simulink model "iot_casestudy_1_32"  (R2023a)
settings: Solver=VariableStepAuto  StartTime=0.0  StopTime=3.0  RelTol=1e-3
undefined symbols (not defined in the file or in its folder): m, n
(part 3 of 3)

== stateflow chart iot_casestudy_1_32/CameraScheduler29 ==
  settings: updateMethod=CONTINUOUS  executeAtInitialization=1
  state Main
    entry:
    dt=timer_array[i];
  (default) -> Main : {i=0;dt=0;}
  Main -> Main : after(dt,msec){i=i+1;send(schedule_driver);send(schedule_control);}
  data: timer_array input; i local double; schedule_driver output double; schedule_control output double; dt local double

== stateflow chart iot_casestudy_1_32/CameraScheduler30 ==
  settings: updateMethod=CONTINUOUS  executeAtInitialization=1
  state Main
    entry:
    dt=timer_array[i];
  (default) -> Main : {i=1;dt=0;}
  Main -> Main : after(dt,msec){i=i+1;send(schedule_driver);send(schedule_control);}
  data: timer_array input; schedule_driver output double; schedule_control output double; dt local double; dt2 local double; i local double =0.0

== stateflow chart iot_casestudy_1_32/CameraScheduler31 ==
  settings: updateMethod=CONTINUOUS  executeAtInitialization=1
  state Main
    entry:
    dt=timer_array[i];
  (default) -> Main : {i=0;dt=0;}
  Main -> Main : after(dt,msec){i=i+1;send(schedule_driver);send(schedule_control);}
  data: timer_array input; i local double; schedule_driver output double; schedule_control output double; dt local double

== stateflow chart iot_casestudy_1_32/CameraDriver ==
  settings: updateMethod=CONTINUOUS
  state Operation
    state CarVisibility [parallel]
      settings: executionOrder=1
      state NoCar
        entry: car=0;
      state Car
        entry: car=1;
      (default) -> NoCar
      NoCar -> Car : [traffic_state==1]
      Car -> NoCar : [traffic_state==0]
    state DriverOperation [parallel]
      settings: executionOrder=2
      state Main
      (default) -> Main : {i=1;}
      Main -> (junction 22) : schedule[image_request]
      (junction 22) -> Main [order 2] : {image.data=0;
          | send(image);i = i + 1;}
      (junction 22) -> Main [order 1] : [(car==1)&&(blurryness(i)==1)]
          | {image.data=1;i = i + 1;send(image);}
  data: image_request input; traffic_state input; blurryness input; image output; car local; i local; schedule input

== stateflow chart iot_casestudy_1_32/CameraControl ==
  settings: updateMethod=CONTINUOUS
  state Operation
    state RequestHangling [parallel]
      settings: executionOrder=1
      state Operation1
      (default) -> Operation1 : {image_request=1;}
      Operation1 -> Operation1 : schedule{image_request=1;}
    state ImageMessaging [parallel]
      settings: executionOrder=2
      state Operation2
        entry:
        validity=isvalid(imageIn);
      (default) -> Operation2 : {i=1;}
      (junction 28) -> Operation2 [order 1] : [validity==1]
          | {receive(imageIn);i = i + 1;
          | imageOut.data=imageIn.data
          | send(imageOut);}
      (junction 28) -> Operation2 [order 2] : {i = i + 1;receive(imageIn);}
      (junction 19) -> (junction 28) [order 1] : [network_faults(i)==0]
      (junction 19) -> Operation2 [order 2] : {receive(imageIn);i = i + 1;}
      Operation2 -> (junction 19) : schedule
  (default) -> Operation
  data: image_request output; imageIn input; i local; network_faults input; imageOut output; schedule input; validity local

== stateflow chart iot_casestudy_1_32/Traffic ==
  settings: updateMethod=CONTINUOUS
  state Nocar
    entry:
    traffic_state=0;
  state Car
    entry:
    traffic_state=1;
  state Nocar1
    entry:
    traffic_state=0;
  (default) -> Nocar
  Nocar -> Car : after(arrive_time,msec)
  Car -> Nocar1 : after(visibility_time,msec)
  data: arrive_time input; visibility_time input; traffic_state output

== stateflow chart iot_casestudy_1_32/Edge ==
  state Waiting
  state NotRecognized
    wait_time=elapsed(msec);
  state Recognized
  (default) -> Waiting : {faults=0;}
  Waiting -> Waiting [order 5] : image3{receive(image3);}
  Waiting -> Waiting [order 3] : image1{receive(image1);}
  Waiting -> Waiting [order 6] : image4{receive(image4);}
  Waiting -> Waiting [order 18] : image17{receive(image17);}
  Waiting -> Waiting [order 19] : image18{receive(image18);}
  Waiting -> Waiting [order 26] : image25{receive(image25);}
  Waiting -> Waiting [order 7] : image5{receive(image5);}
  Waiting -> Waiting [order 9] : image8{receive(image8);}
  Waiting -> Waiting [order 21] : image20{receive(image20);}
  Waiting -> Waiting [order 29] : image28{receive(image28);}
  Waiting -> Waiting [order 20] : image19{receive(image19);}
  Waiting -> Waiting [order 23] : image22{receive(image22);}
  Waiting -> Waiting [order 25] : image24{receive(image24);}
  Waiting -> Waiting [order 2] : image2{receive(image2);}
  Waiting -> Waiting [order 22] : image21{receive(image21);}
  Waiting -> Waiting [order 24] : image23{receive(image23);}
  Waiting -> Waiting [order 32] : image31{receive(image31);}
  Waiting -> Waiting [order 1] : image6{receive(image6);}
  Waiting -> Waiting [order 27] : image26{receive(image26);}
  Waiting -> Waiting [order 33] : image32{receive(image32);}
  Waiting -> Waiting [order 31] : image30{receive(image30);}
  Waiting -> Waiting [order 8] : image7{receive(image7);}
  Waiting -> Waiting [order 28] : image27{receive(image27);}
  Waiting -> Waiting [order 30] : image29{receive(image29);}
  Recognized -> Waiting [order 1] : [traffic_state==0]
  Waiting -> NotRecognized [order 4] : [traffic_state==1]
  NotRecognized -> Waiting [order 1] : [traffic_state==0]
      | {faults=1;}
  Waiting -> Waiting [order 10] : image9{receive(image9);}
  Waiting -> Waiting [order 11] : image10{receive(image10);}
  Waiting -> Waiting [order 12] : image11{receive(image11);}
  Waiting -> Waiting [order 13] : image12{receive(image12);}
  Waiting -> Waiting [order 14] : image13{receive(image13);}
  Waiting -> Waiting [order 15] : image14{receive(image14);}
  Waiting -> Waiting [order 16] : image15{receive(image15);}
  Waiting -> Waiting [order 17] : image16{receive(image16);}
  (junction 279) -> NotRecognized [order 2]
  NotRecognized -> (junction 279) [order 19] : image32
      | {receive(image32);}
  (junction 284) -> NotRecognized [order 2]
  NotRecognized -> (junction 284) [order 18] : image31
      | {receive(image31);}
  (junction 277) -> NotRecognized [order 2]
  NotRecognized -> (junction 277) [order 17] : image30
      | {receive(image30);}
  (junction 276) -> NotRecognized [order 2]
  NotRecognized -> (junction 276) [order 15] : image29
      | {receive(image29);}
  (junction 305) -> NotRecognized [order 2]
  NotRecognized -> (junction 305) [order 13] : image28
      | {receive(image28);}
  (junction 263) -> NotRecognized [order 2]
  NotRecognized -> (junction 263) [order 11] : image27
      | {receive(image27);}
  (junction 303) -> NotRecognized [order 2]
  NotRecognized -> (junction 303) [order 9] : image26
      | {receive(image26);}
  (junction 285) -> NotRecognized [order 2]
  NotRecognized -> (junction 285) [order 7] : image25
      | {receive(image25);}
  (junction 302) -> NotRecognized [order 2]
  NotRecognized -> (junction 302) [order 16] : image24
      | {receive(image24);}
  (junction 297) -> NotRecognized [order 2]
  NotRecognized -> (junction 297) [order 14] : image23
      | {receive(image23);}
  (junction 287) -> NotRecognized [order 2]
  NotRecognized -> (junction 287) [order 12] : image22
      | {receive(image22);}
  (junction 318) -> NotRecognized [order 2]
  NotRecognized -> (junction 318) [order 10] : image21
      | {receive(image21);}
  (junction 264) -> NotRecognized [order 2]
  NotRecognized -> (junction 264) [order 8] : image20
      | {receive(image20);}
  (junction 269) -> NotRecognized [order 2]
  NotRecognized -> (junction 269) [order 6] : image19
      | {receive(image19);}
  (junction 261) -> NotRecognized [order 2]
  NotRecognized -> (junction 261) [order 4] : image18
      | {receive(image18);}
  (junction 272) -> NotRecognized [order 2]
  NotRecognized -> (junction 272) [order 3] : image17
      | {receive(image17);}
  (junction 119) -> NotRecognized [order 2]
  NotRecognized -> (junction 119) [order 5] : image16
      | {receive(image16);}
  (junction 117) -> NotRecognized [order 2]
  NotRecognized -> (junction 117) [order 20] : image15
      | {receive(image15);}
  (junction 106) -> NotRecognized [order 2]
  NotRecognized -> (junction 106) [order 21] : image14
      | {receive(image14);}
  (junction 132) -> NotRecognized [order 2]
  NotRecognized -> (junction 132) [order 22] : image13
      | {receive(image13);}
  (junction 108) -> NotRecognized [order 2]
  NotRecognized -> (junction 108) [order 23] : image12
      | {receive(image12);}
  (junction 113) -> NotRecognized [order 2]
  NotRecognized -> (junction 113) [order 24] : image11
      | {receive(image11);}
  (junction 105) -> NotRecognized [order 2]
  NotRecognized -> (junction 105) [order 25] : image10
      | {receive(image10);}
  (junction 120) -> NotRecognized [order 2]
  NotRecognized -> (junction 120) [order 27] : image9
      | {receive(image9);}
  (junction 64) -> NotRecognized [order 2]
  NotRecognized -> (junction 64) [order 33] : image8
      | {receive(image8);}
  (junction 63) -> NotRecognized [order 2]
  NotRecognized -> (junction 63) [order 32] : image7
      | {receive(image7);}
  (junction 62) -> NotRecognized [order 2]
  NotRecognized -> (junction 62) [order 31] : image6
      | {receive(image6);}
  (junction 61) -> NotRecognized [order 2]
  NotRecognized -> (junction 61) [order 30] : image5
      | {receive(image5);}
  (junction 49) -> NotRecognized [order 2]
  NotRecognized -> (junction 49) [order 29] : image4
      | {receive(image4);}
  (junction 45) -> NotRecognized [order 2]
  NotRecognized -> (junction 45) [order 28] : image3
      | {receive(image3);}
  (junction 22) -> NotRecognized [order 2]
  NotRecognized -> (junction 22) [order 2] : image2
      | {receive(image2);}
  (junction 10) -> NotRecognized [order 2]
  NotRecognized -> (junction 10) [order 26] : image1{receive(image1);}
  (junction 264) -> Recognized [order 1] : [image20.data==1]
  (junction 261) -> Recognized [order 1] : [image18.data==1]
  (junction 49) -> Recognized [order 1] : [image4.data==1]
  (junction 22) -> Recognized [order 1] : [image2.data==1]
  (junction 302) -> Recognized [order 1] : [image24.data==1]
  (junction 287) -> Recognized [order 1] : [image22.data==1]
  (junction 64) -> Recognized [order 1] : [image8.data==1]
  (junction 62) -> Recognized [order 1] : [image6.data==1]
  (junction 279) -> Recognized [order 1] : [image32.data==1]
  (junction 305) -> Recognized [order 1] : [image28.data==1]
  (junction 303) -> Recognized [order 1] : [image26.data==1]
  (junction 119) -> Recognized [order 1] : [image16.data==1]
  (junction 108) -> Recognized [order 1] : [image12.data==1]
  (junction 105) -> Recognized [order 1] : [image10.data==1]
  (junction 277) -> Recognized [order 1] : [image30.data==1]
  (junction 106) -> Recognized [order 1] : [image14.data==1]
  Recognized -> Recognized [order 2] : image17{receive(image17);}
  Recognized -> Recognized [order 29] : image18{receive(image18);}
  Recognized -> Recognized [order 31] : image20{receive(image20);}
  Recognized -> Recognized [order 10] : image25{receive(image25);}
  Recognized -> Recognized [order 30] : image19{receive(image19);}
  Recognized -> Recognized [order 32] : image21{receive(image21);}
  Recognized -> Recognized [order 11] : image24{receive(image24);}
  Recognized -> Recognized [order 3] : image32{receive(image32);}
  Recognized -> Recognized [order 33] : image22{receive(image22);}
  Recognized -> Recognized [order 7] : image28{receive(image28);}
  Recognized -> Recognized [order 4] : image31{receive(image31);}
  Recognized -> Recognized [order 5] : image30{receive(image30);}
  Recognized -> Recognized [order 12] : image23{receive(image23);}
  Recognized -> Recognized [order 9] : image26{receive(image26);}
  Recognized -> Recognized [order 8] : image27{receive(image27);}
  Recognized -> Recognized [order 6] : image29{receive(image29);}
  (junction 10) -> Recognized [order 1] : [image1.data==1]
  (junction 263) -> Recognized [order 1] : [image27.data==1]
  (junction 285) -> Recognized [order 1] : [image25.data==1]
  (junction 297) -> Recognized [order 1] : [image23.data==1]
  (junction 318) -> Recognized [order 1] : [image21.data==1]
  (junction 269) -> Recognized [order 1] : [image19.data==1]
  (junction 272) -> Recognized [order 1] : [image17.data==1]
  (junction 113) -> Recognized [order 1] : [image11.data==1]
  (junction 120) -> Recognized [order 1] : [image9.data==1]
  (junction 63) -> Recognized [order 1] : [image7.data==1]
  (junction 61) -> Recognized [order 1] : [image5.data==1]
  (junction 45) -> Recognized [order 1] : [image3.data==1]
  (junction 284) -> Recognized [order 1] : [image31.data==1]
  (junction 276) -> Recognized [order 1] : [image29.data==1]
  (junction 117) -> Recognized [order 1] : [image15.data==1]
  (junction 132) -> Recognized [order 1] : [image13.data==1]
  Recognized -> Recognized [order 21] : image9{receive(image9);}
  Recognized -> Recognized [order 22] : image10{receive(image10);}
  Recognized -> Recognized [order 23] : image11{receive(image11);}
  Recognized -> Recognized [order 24] : image12{receive(image12);}
  Recognized -> Recognized [order 25] : image13{receive(image13);}
  Recognized -> Recognized [order 26] : image14{receive(image14);}
  Recognized -> Recognized [order 27] : image15{receive(image15);}
  Recognized -> Recognized [order 28] : image16{receive(image16);}
  Recognized -> Recognized [order 17] : image8{receive(image8);}
  Recognized -> Recognized [order 18] : image7{receive(image7);}
  Recognized -> Recognized [order 19] : image6{receive(image6);}
  Recognized -> Recognized [order 20] : image5{receive(image5);}
  Recognized -> Recognized [order 13] : image3{receive(image3);}
  Recognized -> Recognized [order 16] : image4{receive(image4);}
  Recognized -> Recognized [order 14] : image2{receive(image2);}
  Recognized -> Recognized [order 15] : image1{receive(image1);}
  data: traffic_state input; image1 input; faults output; image2 input; wait_time output; image3 input; image4 input; image5 input; image6 input; image7 input; image8 input; image9 input; image10 input; image11 input; image12 input; image13 input; image14 input; image15 input; image16 input; image17 input; image18 input; image19 input; image20 input; image21 input; image22 input; image23 input; image24 input; image25 input; image26 input; image27 input; image28 input; image29 input; image30 input; image31 input; image32 input

== stateflow chart iot_casestudy_1_32/CameraScheduler ==
  settings: updateMethod=CONTINUOUS  executeAtInitialization=1
  state Main
    entry:
    dt=timer_array[i];
  (default) -> Main : {i=1;dt=0;}
  Main -> Main : after(dt,msec){i=i+1;send(schedule_driver);send(schedule_control);}
  data: timer_array input; schedule_driver output double; schedule_control output double; dt local double; dt2 local double; i output double =0.0

== stateflow chart iot_casestudy_1_32/CameraControl1 ==
  settings: updateMethod=CONTINUOUS
  state Operation
    state RequestHangling [parallel]
      settings: executionOrder=1
      note: {image_request=1;}
      state Operation1
      (default) -> Operation1
      Operation1 -> Operation1 : schedule{image_request=1;}
    state ImageMessaging [parallel]
      settings: executionOrder=2
      state Operation2
        entry:
        validity=isvalid(imageIn);
      (default) -> Operation2 : {i=1;}
      (junction 29) -> Operation2 [order 1] : [isvalid(imageIn)==1]
          | {receive(imageIn);i = i + 1;
          | imageOut.data=imageIn.data;
          | send(imageOut);}
      (junction 19) -> Operation2 [order 2] : {receive(imageIn);i = i + 1;}
      Operation2 -> (junction 19) : schedule
      (junction 29) -> Operation2 [order 2] : {i = i + 1;receive(imageIn);}
      (junction 19) -> (junction 29) [order 1] : [network_faults(i)==0]
  (default) -> Operation
  data: image_request output; imageIn input; i local; network_faults input; imageOut output; schedule input; validity local

== stateflow chart iot_casestudy_1_32/CameraDriver1 ==
  settings: updateMethod=CONTINUOUS
  state Operation
    state CarVisibility [parallel]
      settings: executionOrder=1
      state NoCar
        entry: car=0;
      state Car
        entry: car=1;
      (default) -> NoCar
      NoCar -> Car : [traffic_state==1]
      Car -> NoCar : [traffic_state==0]
    state DriverOperation [parallel]
      settings: executionOrder=2
      state Main
      (default) -> Main : {i=1;}
      Main -> (junction 22) : schedule
          | [image_request]
      (junction 22) -> Main [order 1] : [(car==1)&&(blurryness(i)==1)]
          | {image.data=1;send(image);i = i + 1;}
      (junction 22) -> Main [order 2] : {image.data=0;
          | send(image);i = i + 1;}
  data: image_request input; traffic_state input; blurryness input; image output; car local; i local; schedule input

== stateflow chart iot_casestudy_1_32/CameraScheduler1 ==
  settings: updateMethod=CONTINUOUS  executeAtInitialization=1
  state Main
    entry:
    dt=timer_array[i];
  (default) -> Main : {i=0;dt=0;}
  Main -> Main : after(dt,msec){i=i+1;send(schedule_driver);send(schedule_control);}
  data: timer_array input; i local double; schedule_driver output double; schedule_control output double; dt local double

== stateflow chart iot_casestudy_1_32/CameraControl2 ==
  settings: updateMethod=CONTINUOUS
  state Operation
    state RequestHangling [parallel]
      settings: executionOrder=1
      state Operation1
      (default) -> Operation1 : {image_request=1;}
      Operation1 -> Operation1 : schedule{image_request=1;}
    state ImageMessaging [parallel]
      settings: executionOrder=2
      state Operation2
        entry:
        validity=isvalid(imageIn);
      (default) -> Operation2 : {i=1;}
      (junction 28) -> Operation2 [order 1] : [validity==1]
          | {receive(imageIn);i = i + 1;
          | imageOut.data=imageIn.data
          | send(imageOut);}
      (junction 28) -> Operation2 [order 2] : {i = i + 1;receive(imageIn);}
      (junction 19) -> (junction 28) [order 1] : [network_faults(i)==0]
      (junction 19) -> Operation2 [order 2] : {receive(imageIn);i = i + 1;}
      Operation2 -> (junction 19) : schedule
  (default) -> Operation
  data: image_request output; imageIn input; i local; network_faults input; imageOut output; schedule input; validity local

== stateflow chart iot_casestudy_1_32/CameraControl3 ==
  settings: updateMethod=CONTINUOUS
  state Operation
    state RequestHangling [parallel]
      settings: executionOrder=1
      note: {image_request=1;}
      state Operation1
      (default) -> Operation1
      Operation1 -> Operation1 : schedule{image_request=1;}
    state ImageMessaging [parallel]
      settings: executionOrder=2
      state Operation2
        entry:
        validity=isvalid(imageIn);
      (default) -> Operation2 : {i=1;}
      (junction 29) -> Operation2 [order 1] : [isvalid(imageIn)==1]
          | {receive(imageIn);i = i + 1;
          | imageOut.data=imageIn.data;
          | send(imageOut);}
      (junction 19) -> Operation2 [order 2] : {receive(imageIn);i = i + 1;}
      Operation2 -> (junction 19) : schedule
      (junction 29) -> Operation2 [order 2] : {i = i + 1;receive(imageIn);}
      (junction 19) -> (junction 29) [order 1] : [network_faults(i)==0]
  (default) -> Operation
  data: image_request output; imageIn input; i local; network_faults input; imageOut output; schedule input; validity local

== stateflow chart iot_casestudy_1_32/CameraDriver2 ==
  settings: updateMethod=CONTINUOUS
  state Operation
    state CarVisibility [parallel]
      settings: executionOrder=1
      state NoCar
        entry: car=0;
      state Car
        entry: car=1;
      (default) -> NoCar
      NoCar -> Car : [traffic_state==1]
      Car -> NoCar : [traffic_state==0]
    state DriverOperation [parallel]
      settings: executionOrder=2
      state Main
      (default) -> Main : {i=1;}
      Main -> (junction 22) : schedule[image_request]
      (junction 22) -> Main [order 2] : {image.data=0;
          | send(image);i = i + 1;}
      (junction 22) -> Main [order 1] : [(car==1)&&(blurryness(i)==1)]
          | {image.data=1;i = i + 1;send(image);}
  data: image_request input; traffic_state input; blurryness input; image output; car local; i local; schedule input

== stateflow chart iot_casestudy_1_32/CameraDriver3 ==
  settings: updateMethod=CONTINUOUS
  state Operation
    state CarVisibility [parallel]
      settings: executionOrder=1
      state NoCar
        entry: car=0;
      state Car
        entry: car=1;
      (default) -> NoCar
      NoCar -> Car : [traffic_state==1]
      Car -> NoCar : [traffic_state==0]
    state DriverOperation [parallel]
      settings: executionOrder=2
      state Main
      (default) -> Main : {i=1;}
      Main -> (junction 22) : schedule
          | [image_request]
      (junction 22) -> Main [order 1] : [(car==1)&&(blurryness(i)==1)]
          | {image.data=1;send(image);i = i + 1;}
      (junction 22) -> Main [order 2] : {image.data=0;
          | send(image);i = i + 1;}
  data: image_request input; traffic_state input; blurryness input; image output; car local; i local; schedule input

== stateflow chart iot_casestudy_1_32/CameraScheduler2 ==
  settings: updateMethod=CONTINUOUS  executeAtInitialization=1
  state Main
    entry:
    dt=timer_array[i];
  (default) -> Main : {i=1;dt=0;}
  Main -> Main : after(dt,msec){i=i+1;send(schedule_driver);send(schedule_control);}
  data: timer_array input; schedule_driver output double; schedule_control output double; dt local double; dt2 local double; i output double =0.0

== stateflow chart iot_casestudy_1_32/CameraScheduler3 ==
  settings: updateMethod=CONTINUOUS  executeAtInitialization=1
  state Main
    entry:
    dt=timer_array[i];
  (default) -> Main : {i=0;dt=0;}
  Main -> Main : after(dt,msec){i=i+1;send(schedule_driver);send(schedule_control);}
  data: timer_array input; i local double; schedule_driver output double; schedule_control output double; dt local double

== stateflow chart iot_casestudy_1_32/CameraControl4 ==
  settings: updateMethod=CONTINUOUS
  state Operation
    state RequestHangling [parallel]
      settings: executionOrder=1
      state Operation1
      (default) -> Operation1 : {image_request=1;}
      Operation1 -> Operation1 : schedule{image_request=1;}
    state ImageMessaging [parallel]
      settings: executionOrder=2
      state Operation2
        entry:
        validity=isvalid(imageIn);
      (default) -> Operation2 : {i=1;}
      (junction 28) -> Operation2 [order 1] : [validity==1]
          | {receive(imageIn);i = i + 1;
          | imageOut.data=imageIn.data
          | send(imageOut);}
      (junction 28) -> Operation2 [order 2] : {i = i + 1;receive(imageIn);}
      (junction 19) -> (junction 28) [order 1] : [network_faults(i)==0]
      (junction 19) -> Operation2 [order 2] : {receive(imageIn);i = i + 1;}
      Operation2 -> (junction 19) : schedule
  (default) -> Operation
  data: image_request output; imageIn input; i local; network_faults input; imageOut output; schedule input; validity local

== stateflow chart iot_casestudy_1_32/CameraControl5 ==
  settings: updateMethod=CONTINUOUS
  state Operation
    state RequestHangling [parallel]
      settings: executionOrder=1
      note: {image_request=1;}
      state Operation1
      (default) -> Operation1
      Operation1 -> Operation1 : schedule{image_request=1;}
    state ImageMessaging [parallel]
      settings: executionOrder=2
      state Operation2
        entry:
        validity=isvalid(imageIn);
      (default) -> Operation2 : {i=1;}
      (junction 29) -> Operation2 [order 1] : [isvalid(imageIn)==1]
          | {receive(imageIn);i = i + 1;
          | imageOut.data=imageIn.data;
          | send(imageOut);}
      (junction 19) -> Operation2 [order 2] : {receive(imageIn);i = i + 1;}
      Operation2 -> (junction 19) : schedule
      (junction 29) -> Operation2 [order 2] : {i = i + 1;receive(imageIn);}
      (junction 19) -> (junction 29) [order 1] : [network_faults(i)==0]
  (default) -> Operation
  data: image_request output; imageIn input; i local; network_faults input; imageOut output; schedule input; validity local

== stateflow chart iot_casestudy_1_32/CameraControl6 ==
  settings: updateMethod=CONTINUOUS
  state Operation
    state RequestHangling [parallel]
      settings: executionOrder=1
      state Operation1
      (default) -> Operation1 : {image_request=1;}
      Operation1 -> Operation1 : schedule{image_request=1;}
    state ImageMessaging [parallel]
      settings: executionOrder=2
      state Operation2
        entry:
        validity=isvalid(imageIn);
      (default) -> Operation2 : {i=1;}
      (junction 28) -> Operation2 [order 1] : [validity==1]
          | {receive(imageIn);i = i + 1;
          | imageOut.data=imageIn.data
          | send(imageOut);}
      (junction 28) -> Operation2 [order 2] : {i = i + 1;receive(imageIn);}
      (junction 19) -> (junction 28) [order 1] : [network_faults(i)==0]
      (junction 19) -> Operation2 [order 2] : {receive(imageIn);i = i + 1;}
      Operation2 -> (junction 19) : schedule
  (default) -> Operation
  data: image_request output; imageIn input; i local; network_faults input; imageOut output; schedule input; validity local

== stateflow chart iot_casestudy_1_32/CameraControl7 ==
  settings: updateMethod=CONTINUOUS
  state Operation
    state RequestHangling [parallel]
      settings: executionOrder=1
      note: {image_request=1;}
      state Operation1
      (default) -> Operation1
      Operation1 -> Operation1 : schedule{image_request=1;}
    state ImageMessaging [parallel]
      settings: executionOrder=2
      state Operation2
        entry:
        validity=isvalid(imageIn);
      (default) -> Operation2 : {i=1;}
      (junction 29) -> Operation2 [order 1] : [isvalid(imageIn)==1]
          | {receive(imageIn);i = i + 1;
          | imageOut.data=imageIn.data;
          | send(imageOut);}
      (junction 19) -> Operation2 [order 2] : {receive(imageIn);i = i + 1;}
      Operation2 -> (junction 19) : schedule
      (junction 29) -> Operation2 [order 2] : {i = i + 1;receive(imageIn);}
      (junction 19) -> (junction 29) [order 1] : [network_faults(i)==0]
  (default) -> Operation
  data: image_request output; imageIn input; i local; network_faults input; imageOut output; schedule input; validity local

== stateflow chart iot_casestudy_1_32/CameraDriver4 ==
  settings: updateMethod=CONTINUOUS
  state Operation
    state CarVisibility [parallel]
      settings: executionOrder=1
      state NoCar
        entry: car=0;
      state Car
        entry: car=1;
      (default) -> NoCar
      NoCar -> Car : [traffic_state==1]
      Car -> NoCar : [traffic_state==0]
    state DriverOperation [parallel]
      settings: executionOrder=2
      state Main
      (default) -> Main : {i=1;}
      Main -> (junction 22) : schedule[image_request]
      (junction 22) -> Main [order 2] : {image.data=0;
          | send(image);i = i + 1;}
      (junction 22) -> Main [order 1] : [(car==1)&&(blurryness(i)==1)]
          | {image.data=1;i = i + 1;send(image);}
  data: image_request input; traffic_state input; blurryness input; image output; car local; i local; schedule input

== stateflow chart iot_casestudy_1_32/CameraDriver5 ==
  settings: updateMethod=CONTINUOUS
  state Operation
    state CarVisibility [parallel]
      settings: executionOrder=1
      state NoCar
        entry: car=0;
      state Car
        entry: car=1;
      (default) -> NoCar
      NoCar -> Car : [traffic_state==1]
      Car -> NoCar : [traffic_state==0]
    state DriverOperation [parallel]
      settings: executionOrder=2
      state Main
      (default) -> Main : {i=1;}
      Main -> (junction 22) : schedule
          | [image_request]
      (junction 22) -> Main [order 1] : [(car==1)&&(blurryness(i)==1)]
          | {image.data=1;send(image);i = i + 1;}
      (junction 22) -> Main [order 2] : {image.data=0;
          | send(image);i = i + 1;}
  data: image_request input; traffic_state input; blurryness input; image output; car local; i local; schedule input

== stateflow chart iot_casestudy_1_32/CameraDriver6 ==
  settings: updateMethod=CONTINUOUS
  state Operation
    state CarVisibility [parallel]
      settings: executionOrder=1
      state NoCar
        entry: car=0;
      state Car
        entry: car=1;
      (default) -> NoCar
      NoCar -> Car : [traffic_state==1]
      Car -> NoCar : [traffic_state==0]
    state DriverOperation [parallel]
      settings: executionOrder=2
      state Main
      (default) -> Main : {i=1;}
      Main -> (junction 22) : schedule[image_request]
      (junction 22) -> Main [order 2] : {image.data=0;
          | send(image);i = i + 1;}
      (junction 22) -> Main [order 1] : [(car==1)&&(blurryness(i)==1)]
          | {image.data=1;i = i + 1;send(image);}
  data: image_request input; traffic_state input; blurryness input; image output; car local; i local; schedule input

== stateflow chart iot_casestudy_1_32/CameraDriver7 ==
  settings: updateMethod=CONTINUOUS
  state Operation
    state CarVisibility [parallel]
      settings: executionOrder=1
      state NoCar
        entry: car=0;
      state Car
        entry: car=1;
      (default) -> NoCar
      NoCar -> Car : [traffic_state==1]
      Car -> NoCar : [traffic_state==0]
    state DriverOperation [parallel]
      settings: executionOrder=2
      state Main
      (default) -> Main : {i=1;}
      Main -> (junction 22) : schedule
          | [image_request]
      (junction 22) -> Main [order 1] : [(car==1)&&(blurryness(i)==1)]
          | {image.data=1;send(image);i = i + 1;}
      (junction 22) -> Main [order 2] : {image.data=0;
          | send(image);i = i + 1;}
  data: image_request input; traffic_state input; blurryness input; image output; car local; i local; schedule input
